simulink subsystem "Beamform_Single_Array"  (R2019b)
settings: Solver=VariableStepAuto  StartTime=0.0  StopTime=10.0  RelTol=1e-3
settings Model: Creator=toons  LastModifiedBy=toons

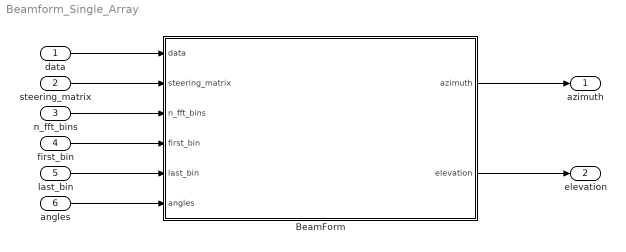
== system Beamform_Single_Array ==
  data : Inport
      settings: VarSizeSig=Yes
  steering_matrix : Inport  Port=2
  n_fft_bins : Inport  Port=3
  first_bin : Inport  Port=4
  last_bin : Inport  Port=5
  angles : Inport  Port=6
  BeamForm : MATLAB Function  TreatAsAtomicUnit=on
  azimuth : Outport
  elevation : Outport  Port=2
  wires:
  angles/1 -> BeamForm/6(angles)
  last_bin/1 -> BeamForm/5(last_bin)
  first_bin/1 -> BeamForm/4(first_bin)
  n_fft_bins/1 -> BeamForm/3(n_fft_bins)
  steering_matrix/1 -> BeamForm/2(steering_matrix)
  data/1 -> BeamForm/1(data)
  BeamForm/1(azimuth) -> azimuth/1
  BeamForm/2(elevation) -> elevation/1

== matlab function Beamform_Single_Array/BeamForm ==
  settings: updateMethod=DISCRETE  sampleTime=BF.model_step
  data: data input size=[BF.batch_size BF.array_size]; steering_matrix input; n_fft_bins input; first_bin input; last_bin input; azimuth output; elevation output; angles input
function [azimuth,elevation] = BeamForm(data, steering_matrix, ...
    n_fft_bins, first_bin, last_bin, angles)
%BEAMFORMDATA Returns the direction of the sound using beamforming.
% Delay & Sum beamforming (FFT is applied in DAS algorithm).

% vector of power per angle
power_angles = zeros(size(steering_matrix,3),1);

% fft of data
dataFFT = fft(data, n_fft_bins); 
% taking only the bins containing the right frequencies
dataFFT = dataFFT(first_bin:last_bin, :);

n_freq = last_bin - first_bin + 1;

% calculating the received power per angle
for freqIt = 1 : n_freq
    % Steering matrix for current frequency bin
    currentA = (squeeze(steering_matrix(:,freqIt,:))'); 

    % Data for current frequency bin
    currentData = (dataFFT(freqIt,:).');

    % Calculating the power for each angle and sum the power to the
    % previous power calculations. We use matrix multiplication to
    % implement the delay and sum beamforming.
    power_angles = power_angles +  abs(currentA * currentData); 
end

[~, max_index] = max(power_angles);
azimuth = angles(1,max_index);
elevation = angles(2,max_index);

end
